simulink model "director"  (R2020a)
settings: Solver=FixedStepAuto  StartTime=0.0  StopTime=inf  FixedStep=0.5  RelTol=1e-3
undefined symbols (not defined in the file): m, n
libraries: robotlib x7
settings Model: EnablePacing=on  Creator=ivory  LastModifiedBy=ivory
settings OptimizationCC: EnhancedBackFolding=on  PassReuseOutputArgsAs=Individual arguments  ZeroExternalMemoryAtStartup=off  ZeroInternalMemoryAtStartup=off  MaxStackSize=64  OptimizeBlockOrder=speed  DifferentSizesBufferReuse=on  OptimizationCustomize=off  EfficientTunableParamExpr=on
settings DebuggingCC: ParameterTunabilityLossMsg=error
settings HardwareCC: ProdBitPerPointer=32  ProdBitPerSizeT=32  ProdBitPerPtrDiffT=32  ProdLargestAtomicFloat=None  ProdIntDivRoundTo=Undefined  ProdEndianess=Unspecified  ProdWordSize=32  ProdHWDeviceType=Generic->Unspecified (assume 32-bit Generic)  UseEmbeddedCoderFeatures=off
settings SFSimCC: MATLABDynamicMemAlloc=off
settings RTWCC: SystemTargetFile=ert.tlc  HardwareBoard=Robot Operating System (ROS)  TemplateMakefile=ert_default_tmf  Toolchain=Catkin  TargetLang=C++
settings CodeAppCC: ForceParamTrailComments=on  IgnoreCustomStorageClasses=off  OperatorAnnotations=on  SimulinkDataObjDesc=on  SFDataObjDesc=on  InsertBlockDesc=on
settings ERTTargetCC: SupportNonInlinedSFcns=on

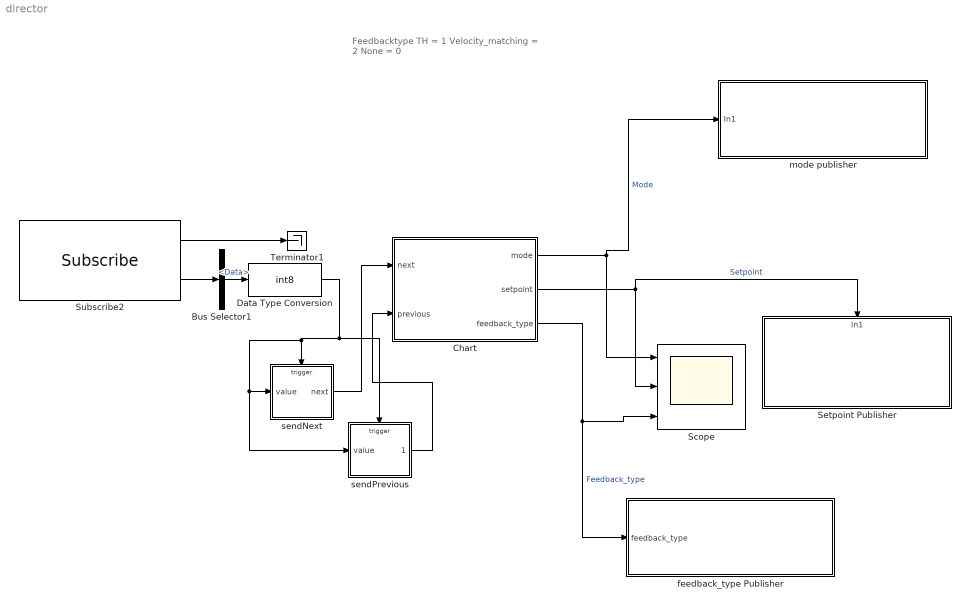
== system director ==
  note: Feedbacktype
      | TH = 1
      | Velocity_matching = 2
      | None = 0
  Bus Selector1 : BusSelector  DialogController=Simulink.DDGSource_BusSelector  OutputSignals=Data
  Chart : Stateflow chart  TreatAsAtomicUnit=on
  Data Type Conversion : DataTypeConversion  OutDataTypeStr=int8
  Scope : Scope  NumInputPorts=3
  Setpoint Publisher : Subsystem
      settings: PortSchema="{\"entries\":[{\"content\":{\"sides\":[{\"content\":{\"connectorIds\":[]},\"type\":\"ConnectorPlacement.EquallySpacedRectSide\",\"uuid\":\"7228cb39-d042-4544-9404-c470f4fdfbf1\"},{\"content\":{\"connectorIds\":[],\"side\":\"RIGHT\"},\"type\":\"ConnectorPlacement.EquallySpacedRectSide\",\"uuid\":\"d3b4c5d4-5a27-4f35-aed9-956300822ff3\"},{\"content\":{\"connectorIds\":[\"In1\"],\"side\":\"TOP\"},\"type\":\"ConnectorPlacement.EquallySpacedRectSide\",\"uuid\":\"960bf3c5-2ad7-4c01-a07e-903e5f41e994\"},{\"content\":{\"connectorIds\":[],\"side\":\"BOTTOM\"},\"type\":\"ConnectorPlacement.EquallySpacedRectSide\",\"uuid\":\"1493639f-9397-4233-abc9-2a06b786f373\"}]},\"type\":\"ConnectorPlacement.EquallySpacedConnector\",\"uuid\":\"6b7d05b9-818d-4613-8d2a-25b4b7d7d80b\"}],\"packageUris\":[\"http://schema.mathworks.com/mf0/Connector/19700101\"],\"version\":\"1.0\"}"
  Subscribe2 : robotlib/Subscribe  topicSource=Specify your own  topic=modeChanger  messageType=std_msgs/Int8  sampleTime=-1  messageQueueLength=1
  Terminator1 : Terminator
  feedback_type Publisher : Subsystem
  mode publisher : Subsystem
  sendNext : Stateflow chart  TreatAsAtomicUnit=on
  sendPrevious : Stateflow chart  TreatAsAtomicUnit=on
  wires:
  Subscribe2/1 -> Terminator1/1
  Subscribe2/2 -> Bus Selector1/1
  Chart/3(feedback_type) -> Scope/3, feedback_type Publisher/1(feedback_type)  "Feedback_type"
  Chart/1(mode) -> mode publisher/1(In1), Scope/1  "Mode"
  Chart/2(setpoint) -> Setpoint Publisher/1(In1), Scope/2  "Setpoint"
  sendNext/1(next) -> Chart/1(next)
  sendPrevious/1(previous) -> Chart/2(previous)
  Data Type Conversion/1 -> sendPrevious/Trigger, sendPrevious/1(value), sendNext/1(value), sendNext/Trigger
  Bus Selector1/1 -> Data Type Conversion/1  "<Data>"

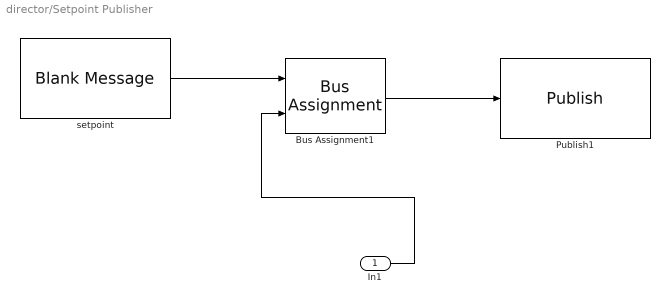
== system director/Setpoint Publisher ==
  In1 : Inport
  Bus Assignment1 : BusAssignment  AssignedSignals=Data
  Publish1 : robotlib/Publish  topicSource=Specify your own  topic=setpoint  messageType=std_msgs/Float64  messageQueueLength=1
  setpoint : robotlib/Blank Message  messageClass=Message  entityType=std_msgs/Float64  messageType=std_msgs/Float64  SampleTime=-1
  wires:
  Bus Assignment1/1 -> Publish1/1
  setpoint/1 -> Bus Assignment1/1
  In1/1 -> Bus Assignment1/2

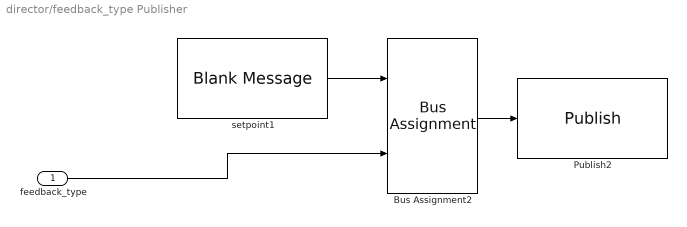
== system director/feedback_type Publisher ==
  feedback_type : Inport
  Bus Assignment2 : BusAssignment  AssignedSignals=Data
  Publish2 : robotlib/Publish  topicSource=Specify your own  topic=feedback_type  messageType=std_msgs/UInt8  messageQueueLength=1
  setpoint1 : robotlib/Blank Message  messageClass=Message  entityType=std_msgs/UInt8  messageType=std_msgs/UInt8  SampleTime=-1
  wires:
  setpoint1/1 -> Bus Assignment2/1
  Bus Assignment2/1 -> Publish2/1
  feedback_type/1 -> Bus Assignment2/2

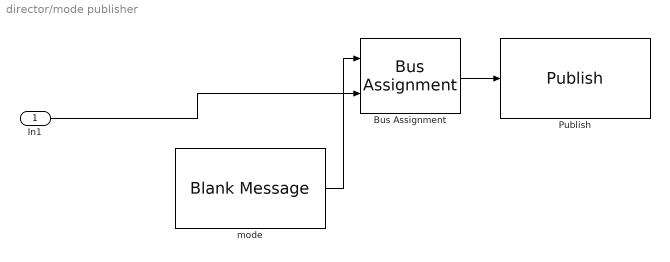
== system director/mode publisher ==
  In1 : Inport
  Bus Assignment : BusAssignment  AssignedSignals=Data
  Publish : robotlib/Publish  topicSource=Specify your own  topic=mode  messageType=std_msgs/UInt8  messageQueueLength=1
  mode : robotlib/Blank Message  messageClass=Message  entityType=std_msgs/UInt8  messageType=std_msgs/UInt8  SampleTime=-1
  wires:
  Bus Assignment/1 -> Publish/1
  mode/1 -> Bus Assignment/1
  In1/1 -> Bus Assignment/2

== stateflow chart director/Chart ==
  state Init
    entry: mode =1;
    setpoint  = 0;
    feedback_type  = 0;
  note: Mode 1 = Drives normally
      | Mode 2 = Constant Time Headway (TH)
      | Mode 3 = Coached Constant TH
      | Mode 4 = Instructed Dynamic TH
      | Mode 5 = Coached Dynamic TH
      | Mode 6 = Instructed Vel Matching
      | Mode 7 = Coached Vel Matching
  state Ghost_mode
    entry: mode = 8;
    setpoint = sp(sp_index); sp_index = sp_index + 1;
    feedback_type = 1;
  state END
  state Instructed_vel_matching
    entry: mode = 6;
    setpoint = 0;
    feedback_type = 0;
  note: Feedbacktype
      | TH = 1
      | Velocity_matching = 2
      | None = 0
  state Coached_dynamic_th
    entry: mode = 5;
    setpoint  = sp(sp_index); sp_index = sp_index + 1;
    feedback_type = 1;
  state Coached_vel_matching
    entry: mode = 7;
    setpoint = 0;
    feedback_type = 2;
  state Const_th
    entry: mode = 2;
    setpoint  = 0;
    feedback_type = 0;
  state Instructed_dynamic_th
    entry: mode = 4;
    setpoint  = sp(sp_index); sp_index = sp_index + 1;
    feedback_type = 0;
  state Coached_const_th
    entry: mode = 3;
    setpoint  = 2.25;
    feedback_type = 1;
    exit: sp_index = 1;
  (default) -> Init [order 1]
  Ghost_mode -> Ghost_mode [order 1] : after(60, sec)[sp_index <=7]
  Instructed_vel_matching -> Init [order 3] : previous
  Init -> Instructed_vel_matching : after(360, sec)
  (default) -> Instructed_vel_matching [order 2] : next
  Ghost_mode -> END [order 2] : [sp_index > 7]
  Coached_dynamic_th -> Ghost_mode [order 2] : next{sp_index = 1;}
  Coached_dynamic_th -> Ghost_mode [order 1] : after(60, sec)[sp_index > 7]{sp_index = 1;}
  Ghost_mode -> Coached_dynamic_th [order 3] : previous{sp_index = 1;}
  Instructed_vel_matching -> Coached_vel_matching [order 2] : next
  Coached_vel_matching -> Instructed_vel_matching [order 3] : previous
  Instructed_vel_matching -> Coached_vel_matching [order 1] : after(360, sec)
  Coached_dynamic_th -> Coached_dynamic_th [order 3] : after(60, sec)[sp_index <=7]
  Instructed_dynamic_th -> Coached_dynamic_th [order 3] : next{sp_index = 1;}
  Instructed_dynamic_th -> Coached_dynamic_th [order 1] : after(60, sec)[sp_index > 7]{sp_index = 1;}
  Coached_dynamic_th -> Instructed_dynamic_th [order 4] : previous{sp_index = 1;}
  Const_th -> Coached_vel_matching [order 3] : previous
  Coached_vel_matching -> Const_th [order 2] : next{sp_index = 1;}
  Coached_vel_matching -> Const_th [order 1] : after(360, sec){sp_index = 1;}
  Instructed_dynamic_th -> Instructed_dynamic_th [order 2] : after(60, sec)[sp_index <=7]
  Coached_const_th -> Instructed_dynamic_th [order 2] : after(360, sec)
  Const_th -> Coached_const_th [order 2] : next
  Coached_const_th -> Const_th [order 3] : previous
  Instructed_dynamic_th -> Coached_const_th [order 4] : previous
  Coached_const_th -> Instructed_dynamic_th [order 1] : next
  Const_th -> Coached_const_th [order 1] : after(360, sec)
  data: mode output uint8; sp constant double size=[1,7] =[2.25, 1.8, 1.35, 1.8, 2.25, 1.35, 2.25]; setpoint output double; sp_index local uint8; feedback_type output uint8; next input; previous input

== stateflow chart director/sendNext ==
  state idle
    during:
    if checkHigh(value)
    next.data = 1;
    send(next)
    end
  (default) -> idle
  data: data function_input; result function_output; next output; value input int8
  events: event input RISING_EDGE_EVENT
  function result = checkHigh(data):
    | function result = checkHigh(data)
    | 
    | if data == 1
    |     result = 1;
    | else
    |     result = 0;
    | end
    | 
    | end

== stateflow chart director/sendPrevious ==
  state idle
    during:
    if checkLow(value)
    previous.data = 1;
    send(previous)
    end
  (default) -> idle
  data: data function_input; result function_output; previous output; value input int8
  events: event input FALLING_EDGE_EVENT
  function result = checkLow(data):
    | function result = checkLow(data)
    | 
    | if data == -1
    |     result = 1;
    | else
    |     result = 0;
    | end
    | 
    | end
